simulink model "sim_noise_reduction"  (R2022a)
settings: Solver=ode4  StartTime=0.0  StopTime=10.0  FixedStep=0.001  RelTol=1e-3
libraries: simulink x1
settings Model: Creator=kawata  LastModifiedBy=kawata
settings SolverCC: AlgebraicLoopSolver=TrustRegion
settings DataIOCC: ReturnWorkspaceOutputs=off
settings DebuggingCC: UnconnectedInputMsg=warning  UnconnectedOutputMsg=warning  UnconnectedLineMsg=warning  SFMachineParentedDataDiag=warning  ArithmeticOperatorsInVariantConditions=warning
settings SFSimCC: SimUseLocalCustomCode=off  CustomCodeUndefinedFunction=UseInterfaceOnly
settings RTWCC: RTWUseLocalCustomCode=off

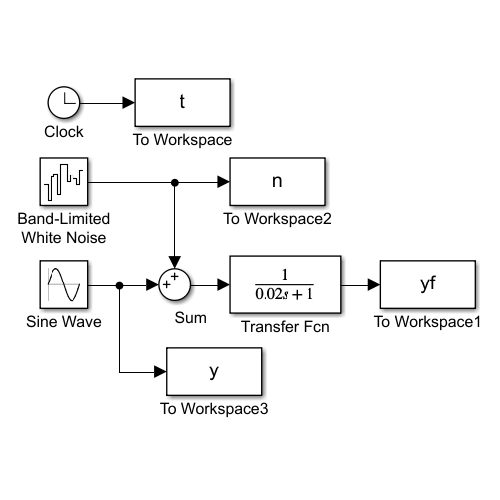
[thumbnail: Simulink's stored preview of the top-level diagram]
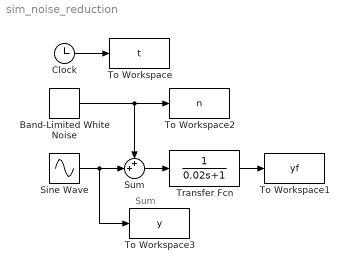
== system sim_noise_reduction ==
  note: Sum
  Band-Limited White Noise : simulink/Sources/Band-Limited White Noise  Cov=[1e-5]  Ts=0.001  seed=[23341]
  Clock : Clock
  Sine Wave : Sin  SampleTime=0
  Sum : Sum  Inputs=++|
  To Workspace : ToWorkspace  VariableName=t  SampleTime=-1
  To Workspace1 : ToWorkspace  VariableName=yf  SampleTime=-1
  To Workspace2 : ToWorkspace  VariableName=n  SampleTime=-1
  To Workspace3 : ToWorkspace  VariableName=y  SampleTime=-1
  Transfer Fcn : TransferFcn  Denominator=[0.02 1]
  wires:
  Sine Wave/1 -> To Workspace3/1, Sum/2
  Sum/1 -> Transfer Fcn/1
  Transfer Fcn/1 -> To Workspace1/1
  Band-Limited White Noise/1 -> To Workspace2/1, Sum/1
  Clock/1 -> To Workspace/1
